simulink model "Drone_PID_rev5_Tuned_Manual_PID"  (R2021b)
settings: Solver=ode5  StartTime=0.0  StopTime=60  FixedStep=1e-2  RelTol=1e-3
values from neighbouring files (symbols this model uses):
  g = robot.env.g    [A_Main.m]
  Kf = robot.aero.Kthrust    [A_Main.m]
  Km = robot.aero.Ktorque    [A_Main.m]
  L = robot.geom.L    [A_Main.m]
  mass = robot.geom.mass*(0.40*rand()-0.20+1)    [A_Main.m]
  maxRPM = robot.rotor.rpm    [A_Main.m]
  T = [Kf                              Kf                             Kf                             Kf ... (first row only)    [A_Main.m]
  Tinv = inv(T)    [A_Main.m]
  Wmax = maxRPM*2*pi/60    [A_Main.m]
undefined symbols (not defined in the file or in its folder): sigbuilder_block
libraries: aerolibconvert2 x5, shared6dof x1
settings Model: Creator=Hassan  LastModifiedBy=Hassan
settings SolverCC: AlgebraicLoopSolver=TrustRegion
settings DebuggingCC: ArithmeticOperatorsInVariantConditions=warning
settings SFSimCC: CustomCodeUndefinedFunction=UseInterfaceOnly
settings CodeAppCC: StateflowObjectComments=on

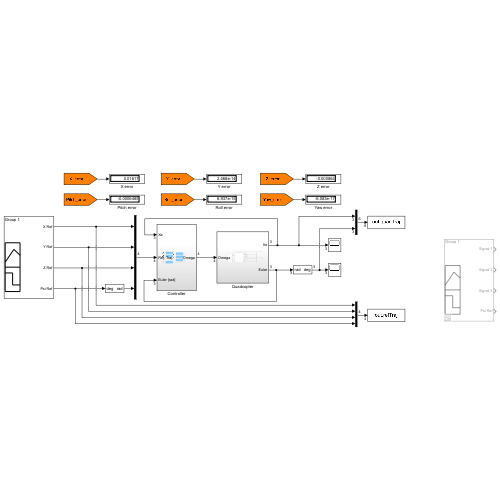
[thumbnail: Simulink's stored preview of the top-level diagram]
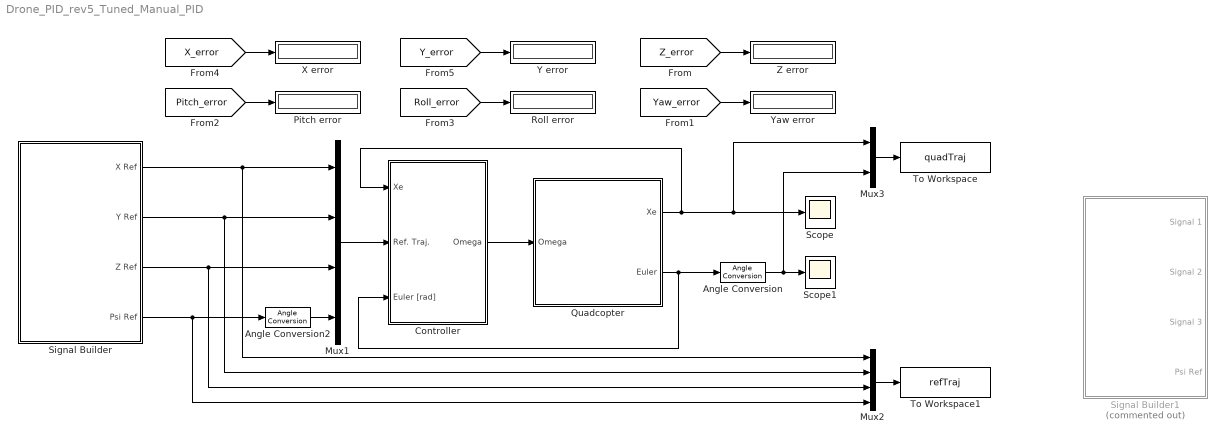
== system Drone_PID_rev5_Tuned_Manual_PID ==
  Angle Conversion : aerolibconvert2/Angle Conversion  IU=rad  OU=deg
  Angle Conversion2 : aerolibconvert2/Angle Conversion  IU=deg  OU=rad
  Controller : Subsystem
  Mux1 : Mux
  Mux2 : Mux
  Mux3 : Mux  Inputs=2
  Pitch error : Display
  Quadcopter : Subsystem
  Roll error : Display
  Scope : Scope
  Scope1 : Scope
  Signal Builder : Subsystem  Tag=STV Subsys  LoadFcn=sigbuilder_block('load');  StartFcn=sigbuilder_block('start');  StopFcn=sigbuilder_block('stop');  ClipboardFcn=sigbuilder_block('clipboard');  mask(Sigbuilder block){tuvar=[0:10]}
      mask help: Simulink:masks:SigbuilderBlock_MD
      mask init:
      | if ~strcmp(get_param(bdroot(gcbh),'SimulationStatus'),'stopped') tuvar = sigbuilder_block('maskInit'); end
      settings: CopyFcn=sigbuilder_block('copy');  DeleteFcn=sigbuilder_block('delete');  ModelCloseFcn=sigbuilder_block('modelClose');  PreSaveFcn=sigbuilder_block('preSave');  PauseFcn=sigbuilder_block('pause');  ContinueFcn=sigbuilder_block('continue');  NameChangeFcn=sigbuilder_block('namechange');  OpenFcn=sigbuilder_block('open',[379.8 118.8 550.8 400.2 ]);  CloseFcn=sigbuilder_block('close');
      mask Display: plot(0, 0, 100, 100,[2, 2, 32, 32, 2], [68, 8, 8, 68, 68],[32, 2], [38, 38], [32, 19, 2],[53, 60, 44], [32, 17, 17, 2],[16, 16, 31, 31]);txt = getActiveGroup(gcbh);text(2, 100, txt,'verticalAlignment', 'top');
  Signal Builder1 : Subsystem  Tag=STV Subsys  Commented=on  LoadFcn=sigbuilder_block('load');  StartFcn=sigbuilder_block('start');  StopFcn=sigbuilder_block('stop');  ClipboardFcn=sigbuilder_block('clipboard');  mask(Sigbuilder block){tuvar=[0:10]}
      mask help: Simulink:masks:SigbuilderBlock_MD
      mask init:
      | if ~strcmp(get_param(bdroot(gcbh),'SimulationStatus'),'stopped') tuvar = sigbuilder_block('maskInit'); end
      settings: CopyFcn=sigbuilder_block('copy');  DeleteFcn=sigbuilder_block('delete');  ModelCloseFcn=sigbuilder_block('modelClose');  PreSaveFcn=sigbuilder_block('preSave');  PauseFcn=sigbuilder_block('pause');  ContinueFcn=sigbuilder_block('continue');  NameChangeFcn=sigbuilder_block('namechange');  OpenFcn=sigbuilder_block('open',[379.8 118.8 550.8 400.2 ]);  CloseFcn=sigbuilder_block('close');
      mask Display: plot(0, 0, 100, 100,[2, 2, 32, 32, 2], [68, 8, 8, 68, 68],[32, 2], [38, 38], [32, 19, 2],[53, 60, 44], [32, 17, 17, 2],[16, 16, 31, 31]);txt = getActiveGroup(gcbh);text(2, 100, txt,'verticalAlignment', 'top');
  To Workspace : ToWorkspace  VariableName=quadTraj  SaveFormat=Timeseries  SampleTime=-1
  To Workspace1 : ToWorkspace  VariableName=refTraj  SaveFormat=Timeseries  SampleTime=-1
  X error : Display
  Y error : Display
  Yaw error : Display
  Z error : Display
  wires:
  [Z_error] -> Z error/1
  Angle Conversion/1 -> Mux3/2, Scope1/1
  [Yaw_error] -> Yaw error/1
  [Pitch_error] -> Pitch error/1
  [Roll_error] -> Roll error/1
  Quadcopter/2(Euler) -> Controller/3(Euler [rad]), Angle Conversion/1
  Quadcopter/1(Xe) -> Mux3/1, Scope/1, Controller/1(Xe)
  Controller/1(Omega) -> Quadcopter/1(Omega)
  [Y_error] -> Y error/1
  [X_error] -> X error/1
  Mux1/1 -> Controller/2("Ref. Traj. ")
  Angle Conversion2/1 -> Mux1/4
  Mux3/1 -> To Workspace/1
  Signal Builder/4(Psi Ref) -> Mux2/4, Angle Conversion2/1
  Signal Builder/3(Z Ref) -> Mux2/3, Mux1/3
  Signal Builder/2(Y Ref) -> Mux2/2, Mux1/2
  Signal Builder/1(X Ref) -> Mux2/1, Mux1/1
  Mux2/1 -> To Workspace1/1

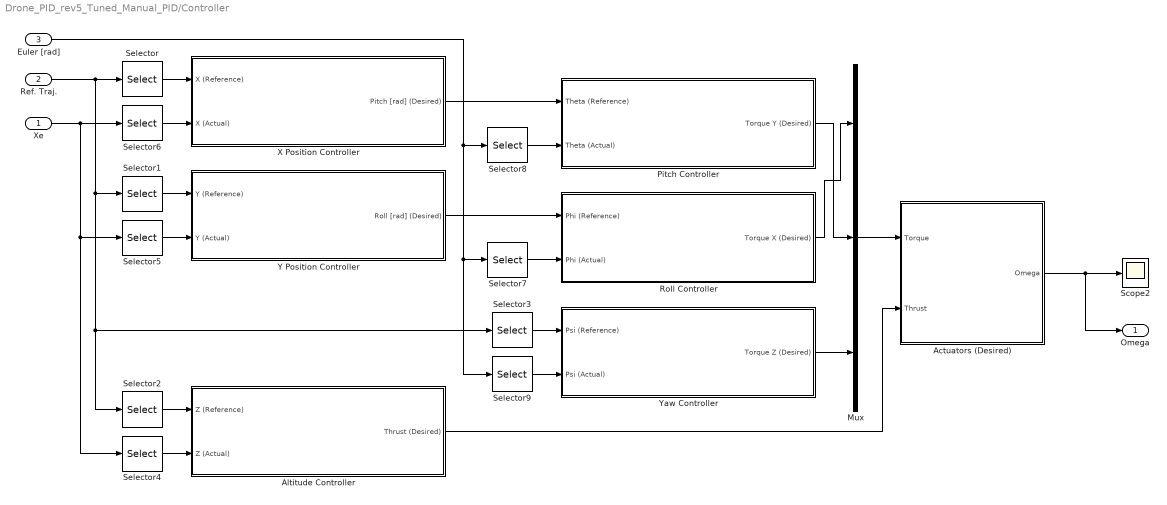
== system Drone_PID_rev5_Tuned_Manual_PID/Controller ==
  Xe : Inport
  "Ref. Traj. " : Inport  Port=2
  Euler [rad] : Inport  Port=3
  Actuators (Desired) : Subsystem
  Altitude Controller : Subsystem
  Mux : Mux  Inputs=3
  Pitch Controller : Subsystem
  Roll Controller : Subsystem
  Scope2 : Scope
  Selector : Selector  InputPortWidth=4  IndexOptions=Index vector (dialog)  Indices=[1]  OutputSizes=1
  Selector1 : Selector  InputPortWidth=4  IndexOptions=Index vector (dialog)  Indices=[2]  OutputSizes=1
  Selector2 : Selector  InputPortWidth=4  IndexOptions=Index vector (dialog)  Indices=[3]  OutputSizes=1
  Selector3 : Selector  InputPortWidth=4  IndexOptions=Index vector (dialog)  Indices=[4]  OutputSizes=1
  Selector4 : Selector  InputPortWidth=3  IndexOptions=Index vector (dialog)  Indices=[3]  OutputSizes=1
  Selector5 : Selector  InputPortWidth=3  IndexOptions=Index vector (dialog)  Indices=[2]  OutputSizes=1
  Selector6 : Selector  InputPortWidth=3  IndexOptions=Index vector (dialog)  Indices=[1]  OutputSizes=1
  Selector7 : Selector  InputPortWidth=3  IndexOptions=Index vector (dialog)  Indices=[1]  OutputSizes=1
  Selector8 : Selector  InputPortWidth=3  IndexOptions=Index vector (dialog)  Indices=[2]  OutputSizes=1
  Selector9 : Selector  InputPortWidth=3  IndexOptions=Index vector (dialog)  Indices=[3]  OutputSizes=1
  X Position Controller : Subsystem
  Y Position Controller : Subsystem
  Yaw Controller : Subsystem
  Omega : Outport  VectorParamsAs1DForOutWhenUnconnected=off
  wires:
  Actuators (Desired)/1(Omega) -> Omega/1, Scope2/1
  Altitude Controller/1(Thrust (Desired)) -> Actuators (Desired)/2(Thrust)
  Mux/1 -> Actuators (Desired)/1(Torque)
  Xe/1 -> Selector4/1, Selector5/1, Selector6/1
  Selector3/1 -> Yaw Controller/1(Psi (Reference))
  Selector/1 -> X Position Controller/1(X (Reference))
  Selector1/1 -> Y Position Controller/1(Y (Reference))
  Selector2/1 -> Altitude Controller/1(Z (Reference))
  "Ref. Traj. "/1 -> Selector2/1, Selector3/1, Selector1/1, Selector/1
  Selector4/1 -> Altitude Controller/2(Z (Actual))
  Selector5/1 -> Y Position Controller/2(Y (Actual))
  Selector6/1 -> X Position Controller/2(X (Actual))
  Selector7/1 -> Roll Controller/2(Phi (Actual))
  Selector8/1 -> Pitch Controller/2(Theta (Actual))
  Selector9/1 -> Yaw Controller/2(Psi (Actual))
  Euler [rad]/1 -> Selector9/1, Selector7/1, Selector8/1
  Yaw Controller/1(Torque Z (Desired)) -> Mux/3
  Pitch Controller/1(Torque Y (Desired)) -> Mux/2
  Roll Controller/1(Torque X (Desired)) -> Mux/1
  X Position Controller/1(Pitch [rad] (Desired)) -> Pitch Controller/1(Theta (Reference))
  Y Position Controller/1(Roll [rad] (Desired)) -> Roll Controller/1(Phi (Reference))

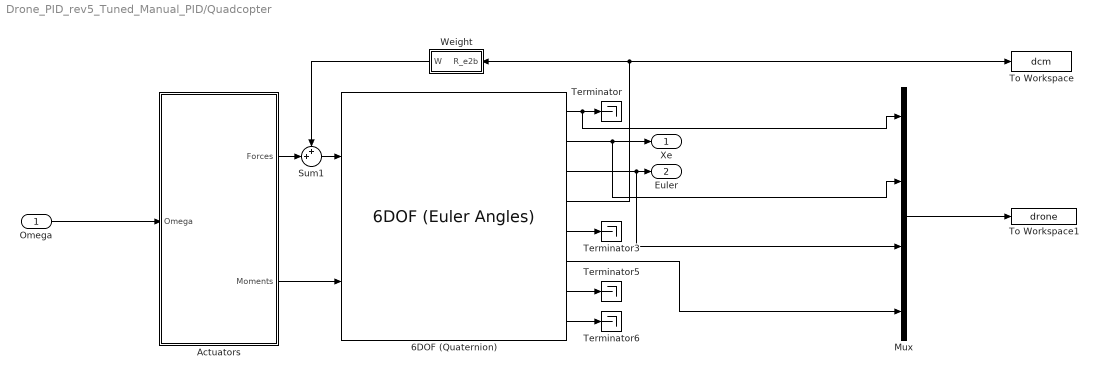
== system Drone_PID_rev5_Tuned_Manual_PID/Quadcopter ==
  Omega : Inport
  6DOF (Quaternion) : shared6dof/6DOF (Euler Angles)  units=Metric (MKS)  mtype=Fixed  rep=Quaternion  xme_0=pos_I_init  Vm_0=vel_B_init  eul_0=euler_I_init  pm_0=angvel_B_init  mass_0=mass  mass_e=0.5  mass_f=2.0  inertia=J  inertia_e=eye(3)  inertia_f=2*eye(3)  k_quat=1.0  vre_flag=on  abi_flag=off  aMode=aMode  xme_statename=''  Vm_statename=''  eul_statename=''  quat_statename=''  pm_statename=''  mass_statename=''
      settings: SourceProductBaseCode=AE,PW,DR,MT,UV,VE
  Actuators : Subsystem
  Mux : Mux
  Sum1 : Sum  Inputs=++|
  Terminator{,3,5..6} (4 alike) : Terminator
  To Workspace : ToWorkspace  VariableName=dcm  SaveFormat=Timeseries  SampleTime=-1
  To Workspace1 : ToWorkspace  VariableName=drone  SaveFormat=Timeseries  SampleTime=-1
  Weight : Subsystem
      mask Display: disp('Weight')
  Xe : Outport  VectorParamsAs1DForOutWhenUnconnected=off
  Euler : Outport  Port=2  VectorParamsAs1DForOutWhenUnconnected=off
  wires:
  6DOF (Quaternion)/1 -> Mux/1, Terminator/1
  6DOF (Quaternion)/8 -> Terminator6/1
  Actuators/1(Forces) -> Sum1/2
  Actuators/2(Moments) -> 6DOF (Quaternion)/2
  6DOF (Quaternion)/7 -> Terminator5/1
  6DOF (Quaternion)/4 -> Weight/1(R_e2b), To Workspace/1
  6DOF (Quaternion)/5 -> Terminator3/1
  6DOF (Quaternion)/6 -> Mux/4
  6DOF (Quaternion)/3 -> Euler/1, Mux/3
  6DOF (Quaternion)/2 -> Mux/2, Xe/1
  Omega/1 -> Actuators/1(Omega)
  Weight/1(W) -> Sum1/1
  Sum1/1 -> 6DOF (Quaternion)/1
  Mux/1 -> To Workspace1/1

== system Drone_PID_rev5_Tuned_Manual_PID/Signal Builder ==
  Demux : Demux  Tag=STV Demux
      settings: DisplayOption=none
  FromWs : FromWorkspace  Tag=STV FromWs  VariableName=tuvar
      SigBuilderData=|
      | common.afterFinalStr = 'Extrapolate'
      | common.sampleTime = 0
      | dataSet.timeRange = [0 60]
      | dataSet.name = 'Group 1'
      | sbobj.Groups.Name = 'Group 1'
      | sbobj.Groups.Signals(1).Name = 'X Ref'
      | sbobj.Groups.Signals(1).XData = [0 0.01 0.02 0.03 0.04 0.05 0.06 0.07 0.08 0.09 0.1 0.11 ... (6001 elements, 1x6001)]
      | sbobj.Groups.Signals(1).YData = [0 0 0 0 0 0 0 0 0 0 0 0 ... (6001 elements, 1x6001)]
      | sbobj.Groups.Signals(2).Name = 'Y Ref'
      | sbobj.Groups.Signals(2).XData = [0 0.01 0.02 0.03 0.04 0.05 0.06 0.07 0.08 0.09 0.1 0.11 ... (6001 elements, 1x6001)]
      | sbobj.Groups.Signals(2).YData = [0 0 0 0 0 0 0 0 0 0 0 0 ... (6001 elements, 1x6001)]
      | sbobj.Groups.Signals(3).Name = 'Z Ref'
      | sbobj.Groups.Signals(3).XData = [0 0.01 0.02 0.03 0.04 0.05 0.06 0.07 0.08 0.09 0.1 0.11 ... (6001 elements, 1x6001)]
      | sbobj.Groups.Signals(3).YData = [0 0 0 0 0 0 0 0 0 0 0 0 ... (6001 elements, 1x6001)]
      | sbobj.Groups.Signals(4).Name = 'Psi Ref'
      | sbobj.Groups.Signals(4).XData = [0 60]
      | sbobj.Groups.Signals(4).YData = [0 0]
      | sbobj.Groups.TimeRange = [0 60]
  X Ref : Outport  Tag=STV Outport
  Y Ref : Outport  Tag=STV Outport  Port=2
  Z Ref : Outport  Tag=STV Outport  Port=3
  Psi Ref : Outport  Tag=STV Outport  Port=4
  wires:
  FromWs/1 -> Demux/1
  Demux/1 -> X Ref/1
  Demux/2 -> Y Ref/1
  Demux/3 -> Z Ref/1
  Demux/4 -> Psi Ref/1

== system Drone_PID_rev5_Tuned_Manual_PID/Signal Builder1 ==
  Demux : Demux  Tag=STV Demux
      settings: DisplayOption=none
  FromWs : FromWorkspace  Tag=STV FromWs  VariableName=tuvar
      SigBuilderData=|
      | common.afterFinalStr = 'Extrapolate'
      | common.sampleTime = 0
      | dataSet.timeRange = [0 60]
      | dataSet.name = 'Group 1'
      | sbobj.Groups.Name = 'Group 1'
      | sbobj.Groups.Signals(1).Name = 'Signal 1'
      | sbobj.Groups.Signals(1).XData = [0 0.01 0.02 0.03 0.04 0.05 0.06 0.07 0.08 0.09 0.1 0.11 ... (6001 elements, 1x6001)]
      | sbobj.Groups.Signals(1).YData = [0 0 0 0 0 0 0 0 0 0 0 0 ... (6001 elements, 1x6001)]
      | sbobj.Groups.Signals(2).Name = 'Signal 2'
      | sbobj.Groups.Signals(2).XData = [0 0.01 0.02 0.03 0.04 0.05 0.06 0.07 0.08 0.09 0.1 0.11 ... (6001 elements, 1x6001)]
      | sbobj.Groups.Signals(2).YData = [0 0 0 0 0 0 0 0 0 0 0 0 ... (6001 elements, 1x6001)]
      | sbobj.Groups.Signals(3).Name = 'Signal 3'
      | sbobj.Groups.Signals(3).XData = [0 0.01 0.02 0.03 0.04 0.05 0.06 0.07 0.08 0.09 0.1 0.11 ... (6001 elements, 1x6001)]
      | sbobj.Groups.Signals(3).YData = [0 0 0 0 0 0 0 0 0 0 0 0 ... (6001 elements, 1x6001)]
      | sbobj.Groups.Signals(4).Name = 'Psi Ref'
      | sbobj.Groups.Signals(4).XData = [0 60]
      | sbobj.Groups.Signals(4).YData = [0 0]
      | sbobj.Groups.TimeRange = [0 60]
  Signal 1 : Outport  Tag=STV Outport
  Signal 2 : Outport  Tag=STV Outport  Port=2
  Signal 3 : Outport  Tag=STV Outport  Port=3
  Psi Ref : Outport  Tag=STV Outport  Port=4
  wires:
  FromWs/1 -> Demux/1
  Demux/1 -> Signal 1/1
  Demux/2 -> Signal 2/1
  Demux/3 -> Signal 3/1
  Demux/4 -> Psi Ref/1

== system Drone_PID_rev5_Tuned_Manual_PID/Controller/Actuators (Desired) ==
  Torque : Inport
  Thrust : Inport  Port=2
  Gain : Gain  Gain=Tinv  Multiplication=Matrix(K*u)
  Limit Omega (rad/sec) due to Motor Constraints : Saturate  UpperLimit=Wmax  LowerLimit=0
  Mux : Mux  Inputs=2
  Sqrt : Sqrt  SaturateOnIntegerOverflow=on
  Omega : Outport  VectorParamsAs1DForOutWhenUnconnected=off
  wires:
  Torque/1 -> Mux/2
  Thrust/1 -> Mux/1
  Limit Omega (rad/sec) due to Motor Constraints/1 -> Omega/1
  Sqrt/1 -> Limit Omega (rad/sec) due to Motor Constraints/1
  Gain/1 -> Sqrt/1
  Mux/1 -> Gain/1

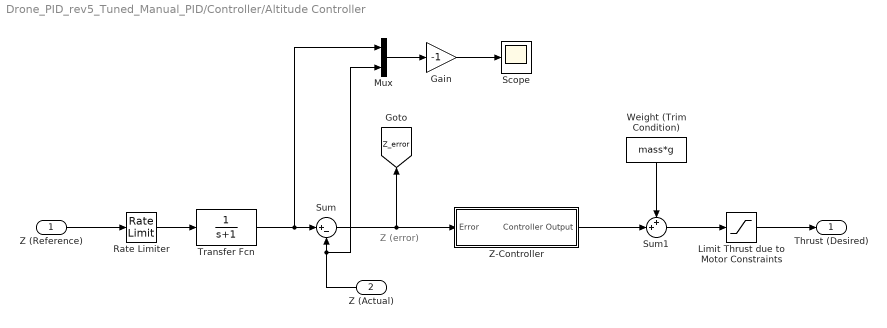
== system Drone_PID_rev5_Tuned_Manual_PID/Controller/Altitude Controller ==
  note: Z (error)
  Z (Reference) : Inport
  Z (Actual) : Inport  Port=2
  Gain : Gain  Gain=-1
  Limit Thrust due to Motor Constraints : Saturate  UpperLimit=4*Kf*(Wmax^2)  LowerLimit=0
  Mux : Mux  Inputs=2
  Rate Limiter : RateLimiter  RisingSlewLimit=2  FallingSlewLimit=-2  SampleTimeMode=inherited
  Scope : Scope
  Sum : Sum  Inputs=|+-
  Sum1 : Sum  Inputs=++|
  Transfer Fcn : TransferFcn  Denominator=[1 1]
  Weight (Trim Condition) : Constant  Value=mass*g
  Z-Controller : Subsystem
  Thrust (Desired) : Outport  VectorParamsAs1DForOutWhenUnconnected=off
  tag scope: Z_error=global
  wires:
  Z-Controller/1(Controller Output) -> Sum1/2
  Weight (Trim Condition)/1 -> Sum1/1
  Sum1/1 -> Limit Thrust due to Motor Constraints/1
  Limit Thrust due to Motor Constraints/1 -> Thrust (Desired)/1
  Mux/1 -> Gain/1
  Z (Reference)/1 -> Rate Limiter/1
  Z (Actual)/1 -> Mux/2, Sum/2
  Gain/1 -> Scope/1
  Transfer Fcn/1 -> Mux/1, Sum/1
  Rate Limiter/1 -> Transfer Fcn/1
  Sum/1 -> Z-Controller/1(Error), [Z_error]

== system Drone_PID_rev5_Tuned_Manual_PID/Controller/Pitch Controller ==
  note: Theta (Error)
  Theta (Reference) : Inport
  Theta (Actual) : Inport  Port=2
  Angle Conversion : aerolibconvert2/Angle Conversion  IU=rad  OU=deg
  Limit Pitch Torque due to Motor Constraints : Saturate  UpperLimit=(Kf*(maxRPM*(2*pi)/60)^2)*L  LowerLimit=-(Kf*(maxRPM*(2*pi)/60)^2)*L
  Mux : Mux  Inputs=2
  Pitch-Controller : Subsystem
  Scope : Scope
  Sum2 : Sum  Inputs=|+-
  Torque Y (Desired) : Outport  VectorParamsAs1DForOutWhenUnconnected=off
  tag scope: Pitch_error=global
  wires:
  Sum2/1 -> [Pitch_error], Pitch-Controller/1(Error)
  Pitch-Controller/1(Controller Output) -> Limit Pitch Torque due to Motor Constraints/1
  Limit Pitch Torque due to Motor Constraints/1 -> Torque Y (Desired)/1
  Angle Conversion/1 -> Scope/1
  Mux/1 -> Angle Conversion/1
  Theta (Actual)/1 -> Mux/2, Sum2/2
  Theta (Reference)/1 -> Mux/1, Sum2/1

== system Drone_PID_rev5_Tuned_Manual_PID/Controller/Roll Controller ==
  note: Phi (Error)
  Phi (Reference) : Inport
  Phi (Actual) : Inport  Port=2
  Angle Conversion : aerolibconvert2/Angle Conversion  IU=rad  OU=deg
  Limit Roll Torque due to Motor Constraints : Saturate  UpperLimit=Kf*(Wmax^2)*L  LowerLimit=-Kf*(Wmax^2)*L
  Mux : Mux  Inputs=2
  Roll-Controller : Subsystem
  Scope : Scope
  Sum2 : Sum  Inputs=|+-
  Torque X (Desired) : Outport  VectorParamsAs1DForOutWhenUnconnected=off
  tag scope: Roll_error=global
  wires:
  Phi (Reference)/1 -> Mux/1, Sum2/1
  Sum2/1 -> [Roll_error], Roll-Controller/1(Error)
  Roll-Controller/1(Controller Output) -> Limit Roll Torque due to Motor Constraints/1
  Limit Roll Torque due to Motor Constraints/1 -> Torque X (Desired)/1
  Mux/1 -> Angle Conversion/1
  Phi (Actual)/1 -> Mux/2, Sum2/2
  Angle Conversion/1 -> Scope/1

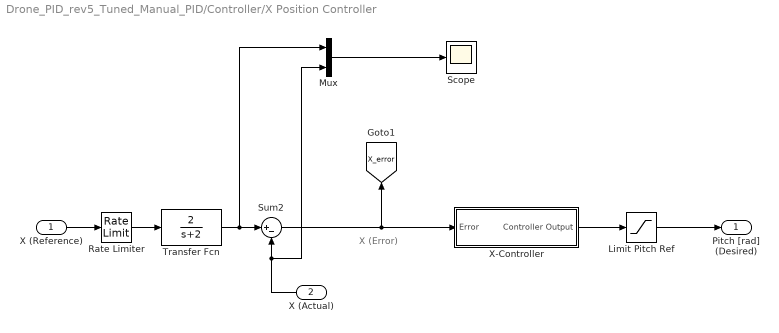
== system Drone_PID_rev5_Tuned_Manual_PID/Controller/X Position Controller ==
  note: X (Error)
  X (Reference) : Inport
  X (Actual) : Inport  Port=2
  Limit Pitch Ref : Saturate  UpperLimit=25*pi/180  LowerLimit=-25*pi/180
  Mux : Mux  Inputs=2
  Rate Limiter : RateLimiter  RisingSlewLimit=3  FallingSlewLimit=-3  SampleTimeMode=inherited
  Scope : Scope
  Sum2 : Sum  Inputs=|+-
  Transfer Fcn : TransferFcn  Numerator=[2]  Denominator=[1 2]
  X-Controller : Subsystem
  Pitch [rad] (Desired) : Outport  VectorParamsAs1DForOutWhenUnconnected=off
  tag scope: X_error=global
  wires:
  Sum2/1 -> [X_error], X-Controller/1(Error)
  X-Controller/1(Controller Output) -> Limit Pitch Ref/1
  Mux/1 -> Scope/1
  X (Reference)/1 -> Rate Limiter/1
  X (Actual)/1 -> Mux/2, Sum2/2
  Limit Pitch Ref/1 -> Pitch [rad] (Desired)/1
  Transfer Fcn/1 -> Mux/1, Sum2/1
  Rate Limiter/1 -> Transfer Fcn/1

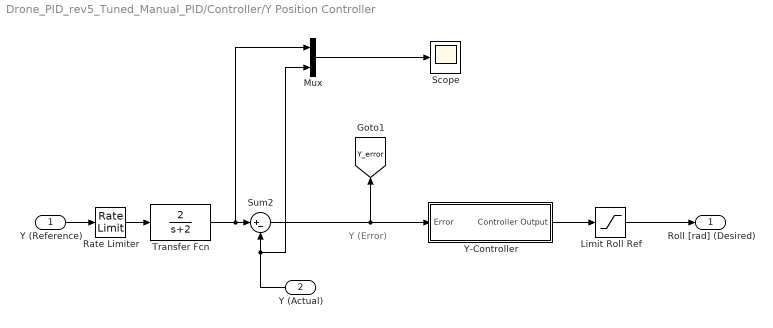
== system Drone_PID_rev5_Tuned_Manual_PID/Controller/Y Position Controller ==
  note: Y (Error)
  Y (Reference) : Inport
  Y (Actual) : Inport  Port=2
  Limit Roll Ref : Saturate  UpperLimit=25*pi/180  LowerLimit=-25*pi/180
  Mux : Mux  Inputs=2
  Rate Limiter : RateLimiter  RisingSlewLimit=3  FallingSlewLimit=-3  SampleTimeMode=inherited
  Scope : Scope
  Sum2 : Sum  Inputs=|+-
  Transfer Fcn : TransferFcn  Numerator=[2]  Denominator=[1 2]
  Y-Controller : Subsystem
  Roll [rad] (Desired) : Outport  VectorParamsAs1DForOutWhenUnconnected=off
  tag scope: Y_error=global
  wires:
  Y (Reference)/1 -> Rate Limiter/1
  Sum2/1 -> Y-Controller/1(Error), [Y_error]
  Y (Actual)/1 -> Mux/2, Sum2/2
  Mux/1 -> Scope/1
  Y-Controller/1(Controller Output) -> Limit Roll Ref/1
  Limit Roll Ref/1 -> Roll [rad] (Desired)/1
  Rate Limiter/1 -> Transfer Fcn/1
  Transfer Fcn/1 -> Mux/1, Sum2/1

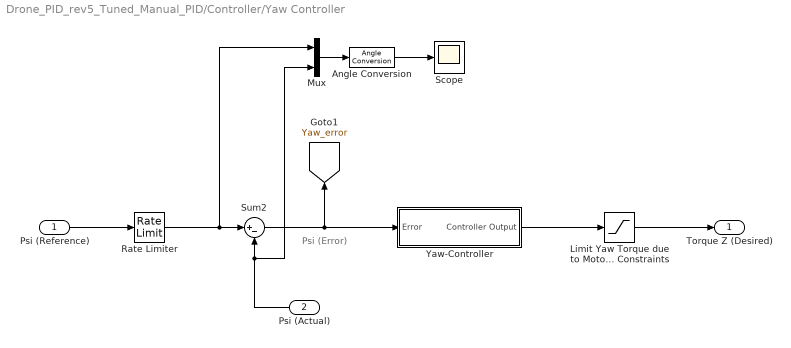
== system Drone_PID_rev5_Tuned_Manual_PID/Controller/Yaw Controller ==
  note: Psi (Error)
  Psi (Reference) : Inport
  Psi (Actual) : Inport  Port=2
  Angle Conversion : aerolibconvert2/Angle Conversion  IU=rad  OU=deg
  Limit Yaw Torque due to Motor Constraints : Saturate  UpperLimit=(Km*(maxRPM*(2*pi)/60)^2)  LowerLimit=-(Km*(maxRPM*(2*pi)/60)^2)
  Mux : Mux  Inputs=2
  Rate Limiter : RateLimiter  RisingSlewLimit=10*pi/180  FallingSlewLimit=-10*pi/180  SampleTimeMode=inherited
  Scope : Scope
  Sum2 : Sum  Inputs=|+-
  Yaw-Controller : Subsystem
  Torque Z (Desired) : Outport  VectorParamsAs1DForOutWhenUnconnected=off
  tag scope: Yaw_error=global
  wires:
  Limit Yaw Torque due to Motor Constraints/1 -> Torque Z (Desired)/1
  Sum2/1 -> Yaw-Controller/1(Error), [Yaw_error]
  Yaw-Controller/1(Controller Output) -> Limit Yaw Torque due to Motor Constraints/1
  Angle Conversion/1 -> Scope/1
  Mux/1 -> Angle Conversion/1
  Psi (Actual)/1 -> Mux/2, Sum2/2
  Psi (Reference)/1 -> Rate Limiter/1
  Rate Limiter/1 -> Mux/1, Sum2/1

== system Drone_PID_rev5_Tuned_Manual_PID/Quadcopter/Actuators ==
  Omega : Inport
  Constant : Constant  Value=0
  Demux : Demux  Outputs=[1 3]
  Gain : Gain  Gain=T  Multiplication=Matrix(K*u)
  Gain1 : Gain  Gain=-1
  Mux : Mux  Inputs=3
  Product : Product
  Forces : Outport  VectorParamsAs1DForOutWhenUnconnected=off
  Moments : Outport  Port=2  VectorParamsAs1DForOutWhenUnconnected=off
  wires:
  Gain/1 -> Demux/1
  Demux/2 -> Moments/1
  Demux/1 -> Gain1/1
  Constant/1 -> Mux/2, Mux/1
  Mux/1 -> Forces/1
  Omega/1 -> Product/2, Product/1
  Product/1 -> Gain/1
  Gain1/1 -> Mux/3

== system Drone_PID_rev5_Tuned_Manual_PID/Quadcopter/Weight ==
  R_e2b : Inport
  Constant1 : Constant  Value=[0 0 g]
  Product : Product  Multiplication=Matrix(*)
  mass : Gain  Gain=mass
  W : Outport  VectorParamsAs1DForOutWhenUnconnected=off
  wires:
  Product/1 -> mass/1
  Constant1/1 -> Product/2
  R_e2b/1 -> Product/1
  mass/1 -> W/1

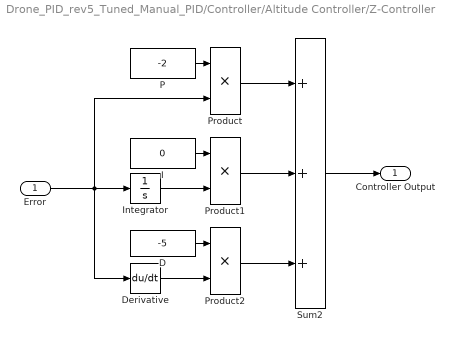
== system Drone_PID_rev5_Tuned_Manual_PID/Controller/Altitude Controller/Z-Controller ==
  Error : Inport
  D : Constant  Value=-5
  Derivative : Derivative
  I : Constant  Value=0
  Integrator : Integrator
  P : Constant  Value=-2
  Product : Product
  Product1 : Product
  Product2 : Product
  Sum2 : Sum  Inputs=+++
  Controller Output : Outport
  wires:
  I/1 -> Product1/1
  Sum2/1 -> Controller Output/1
  Product2/1 -> Sum2/3
  Derivative/1 -> Product2/2
  Product1/1 -> Sum2/2
  Error/1 -> Product/2, Derivative/1, Integrator/1
  P/1 -> Product/1
  Product/1 -> Sum2/1
  Integrator/1 -> Product1/2
  D/1 -> Product2/1

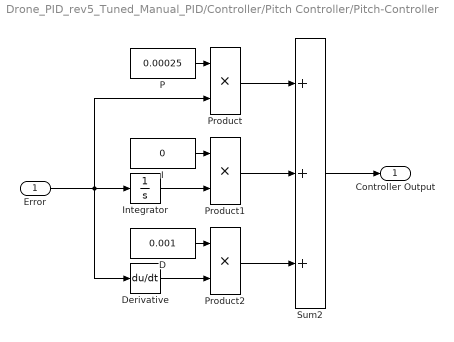
== system Drone_PID_rev5_Tuned_Manual_PID/Controller/Pitch Controller/Pitch-Controller ==
  Error : Inport
  D : Constant  Value=0.001
  Derivative : Derivative
  I : Constant  Value=0
  Integrator : Integrator
  P : Constant  Value=0.00025
  Product : Product
  Product1 : Product
  Product2 : Product
  Sum2 : Sum  Inputs=+++
  Controller Output : Outport
  wires:
  I/1 -> Product1/1
  Sum2/1 -> Controller Output/1
  Product2/1 -> Sum2/3
  Derivative/1 -> Product2/2
  Product1/1 -> Sum2/2
  Error/1 -> Product/2, Derivative/1, Integrator/1
  P/1 -> Product/1
  Product/1 -> Sum2/1
  Integrator/1 -> Product1/2
  D/1 -> Product2/1

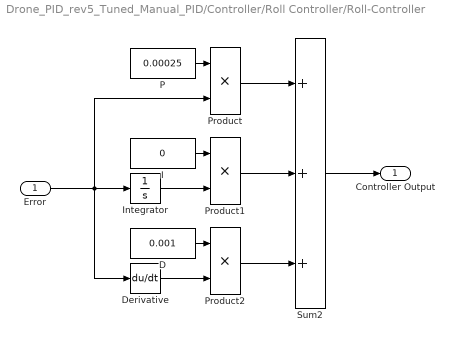
== system Drone_PID_rev5_Tuned_Manual_PID/Controller/Roll Controller/Roll-Controller ==
  Error : Inport
  D : Constant  Value=0.001
  Derivative : Derivative
  I : Constant  Value=0
  Integrator : Integrator
  P : Constant  Value=0.00025
  Product : Product
  Product1 : Product
  Product2 : Product
  Sum2 : Sum  Inputs=+++
  Controller Output : Outport
  wires:
  I/1 -> Product1/1
  Sum2/1 -> Controller Output/1
  Product2/1 -> Sum2/3
  Derivative/1 -> Product2/2
  Product1/1 -> Sum2/2
  Error/1 -> Product/2, Derivative/1, Integrator/1
  P/1 -> Product/1
  Product/1 -> Sum2/1
  Integrator/1 -> Product1/2
  D/1 -> Product2/1

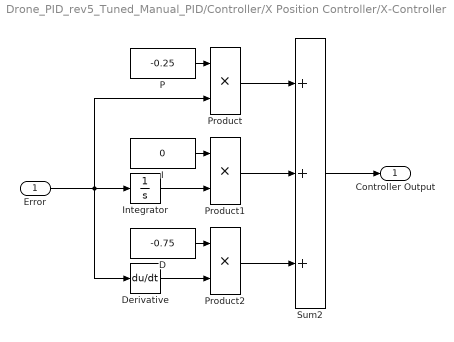
== system Drone_PID_rev5_Tuned_Manual_PID/Controller/X Position Controller/X-Controller ==
  Error : Inport
  D : Constant  Value=-0.75
  Derivative : Derivative
  I : Constant  Value=0
  Integrator : Integrator
  P : Constant  Value=-0.25
  Product : Product
  Product1 : Product
  Product2 : Product
  Sum2 : Sum  Inputs=+++
  Controller Output : Outport
  wires:
  I/1 -> Product1/1
  Sum2/1 -> Controller Output/1
  Product2/1 -> Sum2/3
  Derivative/1 -> Product2/2
  Product1/1 -> Sum2/2
  Error/1 -> Product/2, Derivative/1, Integrator/1
  P/1 -> Product/1
  Product/1 -> Sum2/1
  Integrator/1 -> Product1/2
  D/1 -> Product2/1

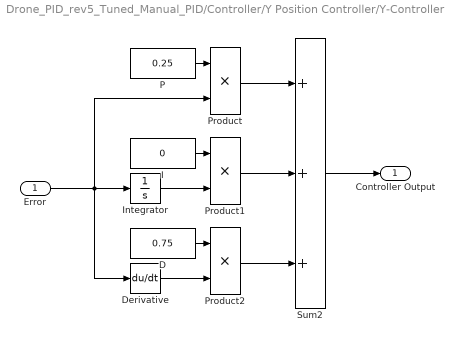
== system Drone_PID_rev5_Tuned_Manual_PID/Controller/Y Position Controller/Y-Controller ==
  Error : Inport
  D : Constant  Value=0.75
  Derivative : Derivative
  I : Constant  Value=0
  Integrator : Integrator
  P : Constant  Value=0.25
  Product : Product
  Product1 : Product
  Product2 : Product
  Sum2 : Sum  Inputs=+++
  Controller Output : Outport
  wires:
  I/1 -> Product1/1
  Sum2/1 -> Controller Output/1
  Product2/1 -> Sum2/3
  Derivative/1 -> Product2/2
  Product1/1 -> Sum2/2
  Error/1 -> Product/2, Derivative/1, Integrator/1
  P/1 -> Product/1
  Product/1 -> Sum2/1
  Integrator/1 -> Product1/2
  D/1 -> Product2/1

== system Drone_PID_rev5_Tuned_Manual_PID/Controller/Yaw Controller/Yaw-Controller ==
  Error : Inport
  D : Constant  Value=0.005
  Derivative : Derivative
  I : Constant  Value=0
  Integrator : Integrator
  P : Constant  Value=0.00175
  Product : Product
  Product1 : Product
  Product2 : Product
  Sum2 : Sum  Inputs=+++
  Controller Output : Outport
  wires:
  I/1 -> Product1/1
  Sum2/1 -> Controller Output/1
  Product2/1 -> Sum2/3
  Derivative/1 -> Product2/2
  Product1/1 -> Sum2/2
  Error/1 -> Product/2, Derivative/1, Integrator/1
  P/1 -> Product/1
  Product/1 -> Sum2/1
  Integrator/1 -> Product1/2
  D/1 -> Product2/1
